simulink model "gyroSakajiri2008Sim"  (R2021b)
settings: Solver=FixedStepAuto  StartTime=0.0  StopTime=final_time  FixedStep=step_time  RelTol=1e-3
values from neighbouring files (symbols this model uses):
  ang_vel_deg = 10    [gyroSakajiri2008.m]
  I0 = 1    [gyroControlDemod.m]    (also in gyroControlPhaseUnmod.m; gyroDigControlDemod.m; gyroModulationsExample.m; gyroSakajiri2008.m)
  mod_amp = (op/2)/mod_sf    (= 0.875)    [gyroControlDemod.m]    (also in gyroControlPhaseUnmod.m; gyroDigControlDemod.m; gyroModulationsExample.m; gyroSakajiri2008.m)
  mod_freq = 1/(4*tau)    (= 54519.689648)    [gyroControlDemod.m]    (also in gyroSakajiri2008.m)
  mod_sf = pi/mod_vpi    (= 0.897597901026)    [gyroControlDemod.m]    (also in gyroControlPhaseUnmod.m; gyroDigControlDemod.m; gyroModulationsExample.m; gyroSakajiri2008.m)
  pd_resp = 1    [gyroControlDemod.m]    (also in gyroControlPhaseUnmod.m; gyroDigControlDemod.m; gyroModulationsExample.m; gyroSakajiri2008.m)
  sf = 2*pi*L*D/(lambda*c)    [gyroControlDemod.m]    (also in gyroControlPhaseUnmod.m; gyroDigControlDemod.m; gyroModulationsExample.m; gyroSakajiri2008.m)
  step_time = tau/10    (= 4.58549932353e-07)    [gyroControlDemod.m]    (also in gyroControlPhaseUnmod.m = 2.29274966176e-06; gyroDigControlDemod.m = 2.29274966176e-06; gyroModulationsExample.m = 4.58549932353e-08; gyroSakajiri2008.m = 1.14637483088e-07)
  tau = L/v    (= 4.58549932353e-06)    [gyroControlDemod.m]    (also in gyroControlPhaseUnmod.m; gyroDigControlDemod.m; gyroModulationsExample.m; gyroSakajiri2008.m)
libraries: dspsigops x2, simulink x1
settings Model: PacingRate=0.001000  Creator=Stinky  LastModifiedBy=Stinky
settings SolverCC: AlgebraicLoopSolver=TrustRegion
settings DebuggingCC: SFMachineParentedDataDiag=warning
settings SFSimCC: SimTargetLang=C++

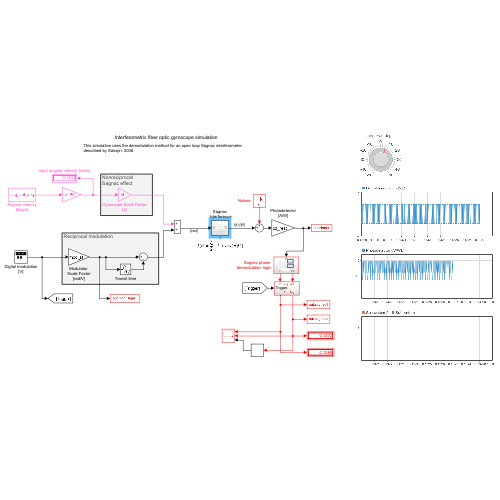
[thumbnail: Simulink's stored preview of the top-level diagram]
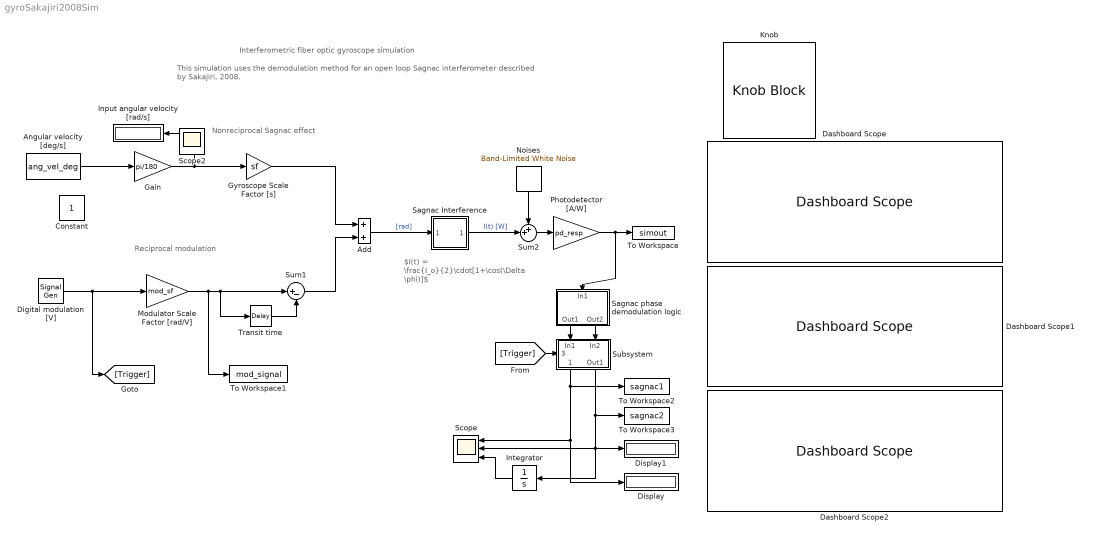
== system gyroSakajiri2008Sim ==
  note: $I(t) = \frac{I_o}{2}\cdot[1+\cos(\Delta \phi)]$
  note: Interferometric fiber optic gyroscope simulation
  note: This simulation uses the demodulation method for an open loop Sagnac interferometer described by Sakajiri, 2008.
  note: Nonreciprocal
      | Sagnac effect
  note: Reciprocal modulation
  Add : Sum
  Angular velocity [deg/s] : Constant  Value=ang_vel_deg
  Dashboard Scope : DashboardScope  TimeSpan=0.001  Ymin=-2  Ymax=2  ScaleAtStop=off  UpdateMode=Scroll
  Dashboard Scope1 : DashboardScope  TimeSpan=0.001  Ymin=-0.2  Ymax=1.2  ScaleAtStop=off
  Dashboard Scope2 : DashboardScope  TimeSpan=0.001
  Digital modulation [V] : SignalGenerator  WaveForm=square  Amplitude=-mod_amp  Frequency=mod_freq
  Display : Display
  Display1 : Display
  Gain : Gain  Gain=pi/180
  Gyroscope Scale Factor [s] : Gain  Gain=sf
  Input angular velocity [rad/s] : Display
  Integrator : Integrator
  Knob : KnobBlock  ScaleMin=-50  ScaleMax=50
  Modulator Scale Factor [rad/V] : Gain  Gain=mod_sf
  Noises : simulink/Sources/Band-Limited White Noise  Cov=1e-14  Ts=step_time  seed=[23341]
  Photodetector [A/W] : Gain  Gain=pd_resp
  Sagnac Interference : Subsystem
  Sagnac phase demodulation logic : Subsystem
  Scope : Scope  NumInputPorts=3
  Subsystem : Subsystem
      settings: PortSchema="{\"entries\":[{\"content\":{\"sides\":[{\"content\":{\"connectorIds\":[\"In1\",\"In2\"]},\"type\":\"ConnectorPlacement.EquallySpacedRectSide\",\"uuid\":\"522e4708-27d0-4988-8289-80d2214b9a62\"},{\"content\":{\"connectorIds\":[\"Out1\",\"Out2\"],\"side\":\"RIGHT\"},\"type\":\"ConnectorPlacement.EquallySpacedRectSide\",\"uuid\":\"5ba00f08-a5b4-4431-b302-217f3991152d\"},{\"content\":{\"connectorIds\":[\"In3\"],\"side\":\"TOP\"},\"type\":\"ConnectorPlacement.EquallySpacedRectSide\",\"uuid\":\"f2cf23db-3373-4eff-b009-f817e854d148\"},{\"content\":{\"connectorIds\":[],\"side\":\"BOTTOM\"},\"type\":\"ConnectorPlacement.EquallySpacedRectSide\",\"uuid\":\"f420c2aa-f197-42ec-8ceb-f7eb675e8f8b\"}]},\"type\":\"ConnectorPlacement.EquallySpacedConnector\",\"uuid\":\"bbc6d32c-1037-4fc8-b2ae-e894be69777a\"}],\"packageUris\":[\"http://schema.mathworks.com/mf0/Connector/R2020b\"],\"version\":\"1.0\"}"
  Sum1 : Sum  Inputs=|+-
  Sum2 : Sum  Inputs=++|
  To Workspace : ToWorkspace  VariableName=simout  SaveFormat=Timeseries  SampleTime=-1
  To Workspace1 : ToWorkspace  VariableName=mod_signal  SaveFormat=Timeseries  SampleTime=-1
  To Workspace2 : ToWorkspace  VariableName=sagnac1  SaveFormat=Timeseries  SampleTime=-1
  To Workspace3 : ToWorkspace  VariableName=sagnac2  SaveFormat=Timeseries  SampleTime=-1
  Transit time : TransportDelay  DelayTime=tau
  Constant : Constant  IOType=siggen
  Scope2 : Scope
  wires:
  Gyroscope Scale Factor [s]/1 -> Add/1
  Add/1 -> Sagnac Interference/1(In1)  "[rad]"
  Transit time/1 -> Sum1/2
  Angular velocity [deg/s]/1 -> Gain/1
  Modulator Scale Factor [rad/V]/1 -> Sum1/1, Transit time/1, To Workspace1/1
  Photodetector [A/W]/1 -> To Workspace/1, Sagnac phase demodulation logic/1(In1)
  Sum2/1 -> Photodetector [A/W]/1
  Sagnac Interference/1(Out1) -> Sum2/2  "I(t) [W]"
  Noises/1 -> Sum2/1
  Sum1/1 -> Add/2
  Sagnac phase demodulation logic/1(Out1) -> Subsystem/1(In1)
  Sagnac phase demodulation logic/2(Out2) -> Subsystem/2(In2)
  Digital modulation [V]/1 -> Modulator Scale Factor [rad/V]/1, [Trigger]
  Subsystem/1(" ") -> Display/1, Scope/1, To Workspace2/1
  Gain/1 -> Gyroscope Scale Factor [s]/1, Input angular velocity [rad/s]/1
  Subsystem/2(Out1) -> Display1/1, Integrator/1, Scope/2, To Workspace3/1
  Integrator/1 -> Scope/3
  [Trigger] -> Subsystem/3(Trigger)

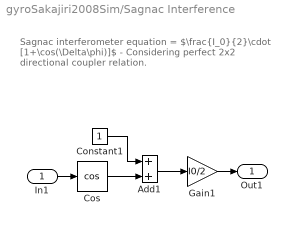
== system gyroSakajiri2008Sim/Sagnac Interference ==
  note: Sagnac interferometer equation = $\frac{I_0}{2}\cdot [1+\cos(\Delta\phi)]$
      |
      | - Considering perfect 2x2 directional coupler relation.
  In1 : Inport
  Add1 : Sum
  Constant1 : Constant
  Cos : Trigonometry  Operator=cos
  Gain1 : Gain  Gain=I0/2
  Out1 : Outport
  wires:
  Add1/1 -> Gain1/1
  Constant1/1 -> Add1/1
  Cos/1 -> Add1/2
  Gain1/1 -> Out1/1
  In1/1 -> Cos/1

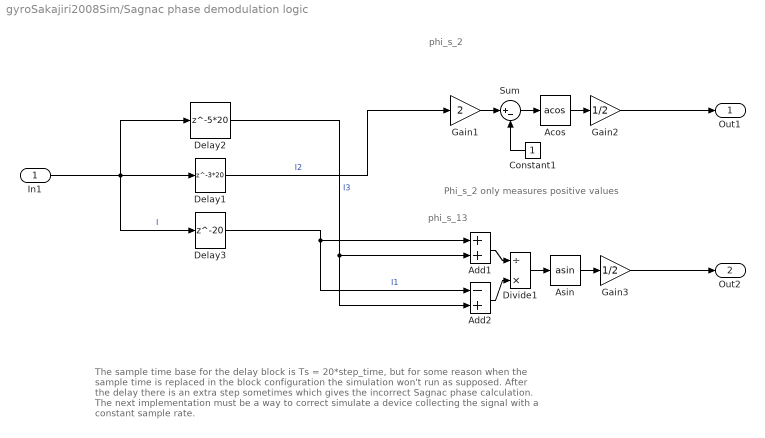
== system gyroSakajiri2008Sim/Sagnac phase demodulation logic ==
  note: Phi_s_2 only measures positive values
  note: The sample time base for the delay block is Ts = 20*step_time,
      | but for some reason when the sample time is replaced in the block
      | configuration the simulation won't run as supposed.
      | After the delay there is an extra step sometimes which gives the incorrect
      | Sagnac phase calculation.
      |
      | The next implementation must be a way to correct simulate a device collecting the signal with a constant sample rate.
  note: phi_s_13
  note: phi_s_2
  In1 : Inport
  Acos : Trigonometry  Operator=acos
  Add1 : Sum
  Add2 : Sum  Inputs=-+
  Asin : Trigonometry  Operator=asin
  Constant1 : Constant
  Delay1 : Delay  DelayLength=3*20
  Delay2 : Delay  DelayLength=5*20
  Delay3 : Delay  DelayLength=20
  Divide1 : Product  Inputs=/*
  Gain1 : Gain  Gain=2
  Gain2 : Gain  Gain=1/2
  Gain3 : Gain  Gain=1/2
  Sum : Sum  Inputs=|+-
  Out1 : Outport
  Out2 : Outport  Port=2
  wires:
  Sum/1 -> Acos/1
  Constant1/1 -> Sum/2
  Delay1/1 -> Gain1/1  "I2"
  Gain3/1 -> Out2/1
  Delay2/1 -> Add1/2, Add2/2  "I3"
  Asin/1 -> Gain3/1
  Acos/1 -> Gain2/1
  Gain1/1 -> Sum/1
  Divide1/1 -> Asin/1
  Gain2/1 -> Out1/1
  Add1/1 -> Divide1/1
  Add2/1 -> Divide1/2
  Delay3/1 -> Add1/1, Add2/1  "I1"
  In1/1 -> Delay3/1, Delay2/1, Delay1/1  "I"

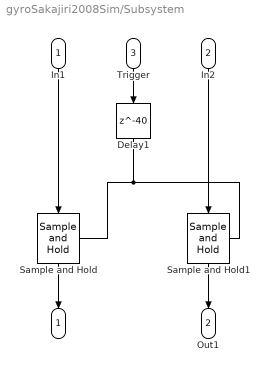
== system gyroSakajiri2008Sim/Subsystem ==
  In1 : Inport
  In2 : Inport  Port=2
  Trigger : Inport  Port=3
  Delay1 : Delay  DelayLength=40
  Sample and Hold : dspsigops/Sample and Hold  trig=Rising edge  initCond=0  latchinput=off
  Sample and Hold1 : dspsigops/Sample and Hold  trig=Rising edge  initCond=0  latchinput=off
  " " : Outport
  Out1 : Outport  Port=2
  wires:
  Sample and Hold1/1 -> Out1/1
  Sample and Hold/1 -> " "/1
  In1/1 -> Sample and Hold/1
  Delay1/1 -> Sample and Hold/Trigger, Sample and Hold1/Trigger
  Trigger/1 -> Delay1/1
  In2/1 -> Sample and Hold1/1
